simulink model "altitudeYawControl"  (R2014a)
settings: Solver=FixedStepDiscrete  SolverMode=SingleTasking  StartTime=0.0  StopTime=10.0  RelTol=1e-3
libraries: arduinolib x3, SkywardBLIMP x2, simulink x1
settings Model: ExtModeTrigDuration=2  Creator=Francescodario  LastModifiedBy=Francescodario
settings OptimizationCC: OptimizeModelRefInitCode=on  LifeSpan=1
settings DebuggingCC: UnderspecifiedInitializationDetection=Classic  SolverPrmCheckMsg=none
settings HardwareCC: ProdBitPerInt=16  ProdBitPerPointer=8  ProdIntDivRoundTo=Zero  ProdEndianess=LittleEndian  ProdWordSize=8  ProdHWDeviceType=Atmel->AVR
settings RTWCC: SystemTargetFile=realtime.tlc  GenerateMakefile=off  TemplateMakefile=realtime.tmf  Description=Run on Target Hardware  RTWVerbose=off  ProcessScript=realtime_make_rtw_hook
settings STFCustomTargetCC: TargetLibSuffix=.a  GenerateSampleERTMain=on  ConcurrentExecutionCompliant=off  GeneratePreprocessorConditionals=Use local settings  ERTCustomFileBanners=on  SupportNonInlinedSFcns=off  SupportVariableSizeSignals=on  MATLABClassNameForMDSCustomization=Simulink.SoftwareTarget.ERTCustomization  GRTInterface=off  SystemTargetFile=realtime.tlc
settings ERTTargetCC: CombineOutputUpdateFcns=off  SupportContinuousTime=on  SupportVariableSizeSignals=on  ExtModeTransport=3  ExtModeMexFile=ext_serial_win32_comm  ExtModeMexArgs=0 1 9600  ERTSrcFileBannerTemplate=realtime_code_template.cgt  ERTHdrFileBannerTemplate=realtime_code_template.cgt  ERTDataSrcFileTemplate=realtime_code_template.cgt  ERTDataHdrFileTemplate=realtime_code_template.cgt  ERTCustomFileTemplate=realtime_file_process.tlc

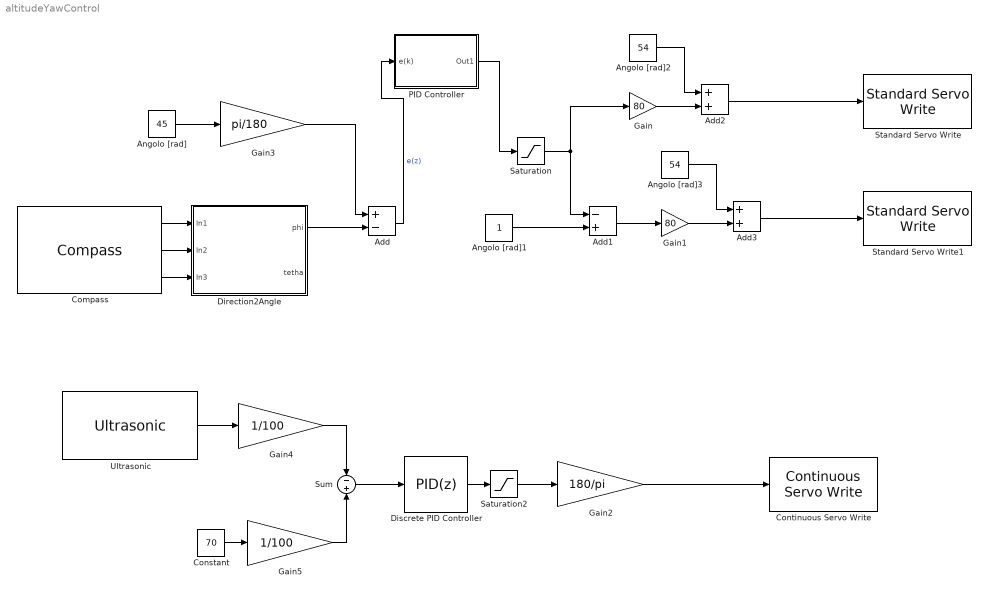
== system altitudeYawControl ==
  Add : Sum  Inputs=+-
  Add1 : Sum  Inputs=-+
  Add2 : Sum
  Add3 : Sum
  Angolo [rad] : Constant  Value=45
  Angolo [rad]1 : Constant
  Angolo [rad]2 : Constant  Value=54
  Angolo [rad]3 : Constant  Value=54
  Compass : SkywardBLIMP/Compass
  Constant : Constant  Value=70
  Continuous Servo Write : arduinolib/Continuous Servo Write  pinNumber=5
      link override Constant: Value=90
  Direction2Angle : Subsystem
  Discrete PID Controller : simulink/Continuous/PID Controller  Controller=PID  TimeDomain=Discrete-time  SampleTime=0.1  IntegratorMethod=Trapezoidal  FilterMethod=Forward Euler  Form=Parallel  P=1.2  I=0.1  D=2  N=0  InitialConditionSource=internal  InitialConditionForIntegrator=0  InitialConditionForFilter=0  ExternalReset=none  LimitOutput=off  UpperSaturationLimit=inf  LowerSaturationLimit=-inf  LinearizeAsGain=off  AntiWindupMode=none  Kb=1  TrackingMode=off  Kt=1  PParamMin=[]  PParamMax=[]  IParamMin=[]  IParamMax=[]  DParamMin=[]  DParamMax=[]  NParamMin=[]  NParamMax=[]  KbParamMin=[]  KbParamMax=[]  KtParamMin=[]  KtParamMax=[]  POutMin=[]  POutMax=[]  IOutMin=[]  IOutMax=[]  DOutMin=[]  DOutMax=[]  NOutMin=[]  NOutMax=[]  KbOutMin=[]  KbOutMax=[]  KtOutMin=[]  KtOutMax=[]  IntegratorOutMin=[]  IntegratorOutMax=[]  FilterOutMin=[]  FilterOutMax=[]  SumOutMin=[]  SumOutMax=[]  SumI1OutMin=[]  SumI1OutMax=[]  SumI2OutMin=[]  SumI2OutMax=[]  SumI3OutMin=[]  SumI3OutMax=[]  SumDOutMin=[]  SumDOutMax=[]  SaturationOutMin=[]  SaturationOutMax=[]  IntegratorContinuousStateAttributes=''  IntegratorStateMustResolveToSignalObject=off  IntegratorRTWStateStorageClass=Auto  FilterContinuousStateAttributes=''  FilterStateMustResolveToSignalObject=off  FilterRTWStateStorageClass=Auto
  Gain : Gain  Gain=80
  Gain1 : Gain  Gain=80
  Gain2 : Gain  Gain=180/pi  SampleTime=0.1
  Gain3 : Gain  Gain=pi/180  SampleTime=0.1
  Gain4 : Gain  Gain=1/100  SampleTime=0.1
  Gain5 : Gain  Gain=1/100  SampleTime=0.1
  PID Controller : Subsystem  mask{Ts=0.5, kp=1.5, ki=0.2, kd=2}
      mask prompts: Ts "Sample Time"; kp "Guadagno Proporzionale"; ki "Guadagno Integrativo"; kd "Guadagno Derivativo"
      mask init:
      | s1=['kp= ',num2str(kp)];
      | s2=['ki= ',num2str(ki)];
      | s3=['kd= ',num2str(kd)];
      | s=strvcat(s1,s2,s3);  %sto concatenando verticalmente
      mask Display: disp(s)
  Saturation : Saturate  UpperLimit=1  LowerLimit=0
  Saturation2 : Saturate  UpperLimit=0.3  LowerLimit=-0.3
  Standard Servo Write : arduinolib/Standard Servo Write  pinNumber=7
  Standard Servo Write1 : arduinolib/Standard Servo Write  pinNumber=4
  Sum : Sum  Inputs=-+
  Ultrasonic : SkywardBLIMP/Ultrasonic
  wires:
  Compass/1 -> Direction2Angle/1(In1)
  Compass/2 -> Direction2Angle/2(In2)
  Compass/3 -> Direction2Angle/3(In3)
  Saturation/1 -> Add1/1, Gain/1
  Add1/1 -> Gain1/1
  Direction2Angle/1(phi) -> Add/2
  Angolo [rad]/1 -> Gain3/1
  Angolo [rad]1/1 -> Add1/2
  Add/1 -> PID Controller/1(e(k))  "e(z)"
  PID Controller/1(Out1) -> Saturation/1
  Gain/1 -> Add2/2
  Angolo [rad]2/1 -> Add2/1
  Gain1/1 -> Add3/2
  Angolo [rad]3/1 -> Add3/1
  Add2/1 -> Standard Servo Write/1
  Add3/1 -> Standard Servo Write1/1
  Constant/1 -> Gain5/1
  Sum/1 -> Discrete PID Controller/1
  Gain2/1 -> Continuous Servo Write/1
  Discrete PID Controller/1 -> Saturation2/1
  Saturation2/1 -> Gain2/1
  Ultrasonic/1 -> Gain4/1
  Gain3/1 -> Add/1
  Gain4/1 -> Sum/1
  Gain5/1 -> Sum/2

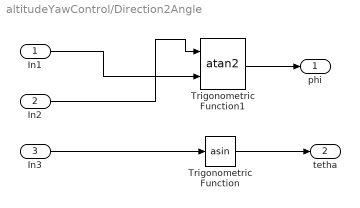
== system altitudeYawControl/Direction2Angle ==
  In1 : Inport
  In2 : Inport  Port=2
  In3 : Inport  Port=3
  Trigonometric Function : Trigonometry  Operator=asin
  Trigonometric Function1 : Trigonometry  Operator=atan2
  phi : Outport
  tetha : Outport  Port=2
  wires:
  In1/1 -> Trigonometric Function1/2
  Trigonometric Function1/1 -> phi/1
  In3/1 -> Trigonometric Function/1
  In2/1 -> Trigonometric Function1/1
  Trigonometric Function/1 -> tetha/1

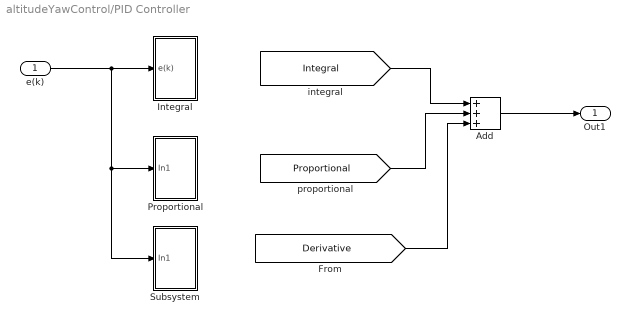
== system altitudeYawControl/PID Controller ==
  e(k) : Inport
  Add : Sum  Inputs=+++
  Integral : Subsystem
  Proportional : Subsystem
  Subsystem : Subsystem
  Out1 : Outport
  wires:
  [Integral] -> Add/1
  Add/1 -> Out1/1
  [Proportional] -> Add/2
  e(k)/1 -> Subsystem/1(In1), Proportional/1(In1), Integral/1(e(k))
  [Derivative] -> Add/3

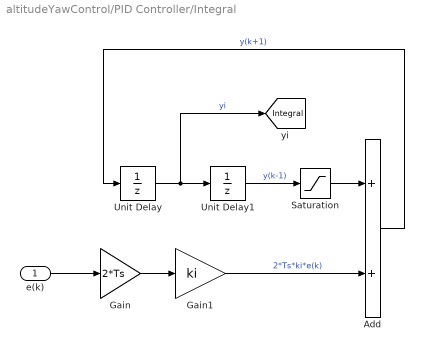
== system altitudeYawControl/PID Controller/Integral ==
  e(k) : Inport
  Add : Sum
  Gain : Gain  Gain=2*Ts
  Gain1 : Gain  Gain=ki
  Saturation : Saturate  UpperLimit=1  LowerLimit=-1
      settings: AttributesFormatString=|
      | %<LowerLimit>
      | %<UpperLimit>
  Unit Delay : UnitDelay  SampleTime=Ts
  Unit Delay1 : UnitDelay  SampleTime=Ts
  tag scope: Integral=global
  wires:
  Gain1/1 -> Add/2  "2*Ts*ki*e(k)"
  Unit Delay/1 -> [Integral], Unit Delay1/1  "yi"
  Gain/1 -> Gain1/1
  Saturation/1 -> Add/1
  Unit Delay1/1 -> Saturation/1  "y(k-1)"
  e(k)/1 -> Gain/1
  Add/1 -> Unit Delay/1  "y(k+1)"

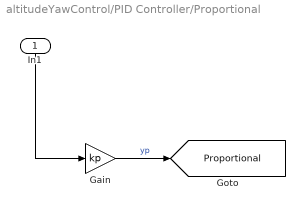
== system altitudeYawControl/PID Controller/Proportional ==
  In1 : Inport
  Gain : Gain  Gain=kp
  tag scope: Proportional=global
  wires:
  Gain/1 -> [Proportional]  "yp"
  In1/1 -> Gain/1

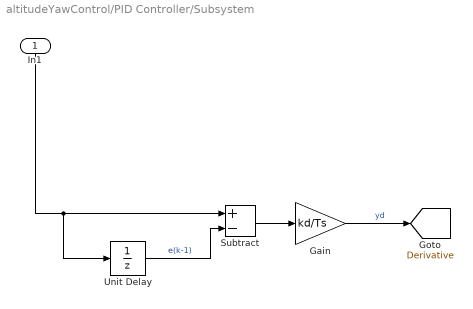
== system altitudeYawControl/PID Controller/Subsystem ==
  In1 : Inport
  Gain : Gain  Gain=kd/Ts
  Subtract : Sum  Inputs=+-
  Unit Delay : UnitDelay  SampleTime=-1
  tag scope: Derivative=global
  wires:
  Unit Delay/1 -> Subtract/2  "e(k-1)"
  Gain/1 -> [Derivative]  "yd"
  Subtract/1 -> Gain/1
  In1/1 -> Unit Delay/1, Subtract/1
